simulink model "sim_qn6a"  (R2022b)
settings: Solver=ode4  StartTime=0.0  StopTime=8.0  FixedStep=tstep  RelTol=1e-3
undefined symbols (not defined in the file): den, num
settings Model: Creator=dipte  LastModifiedBy=dipte
settings DataIOCC: ReturnWorkspaceOutputs=off

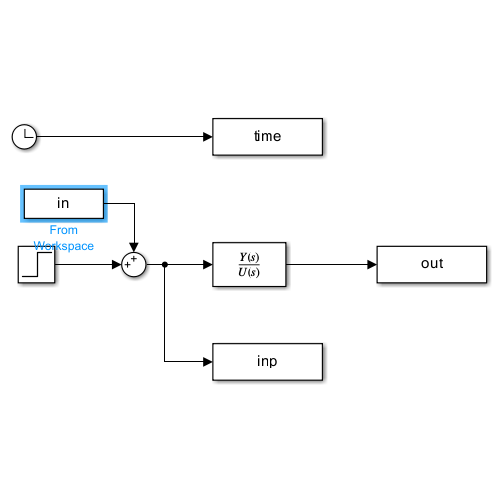
[thumbnail: Simulink's stored preview of the top-level diagram]
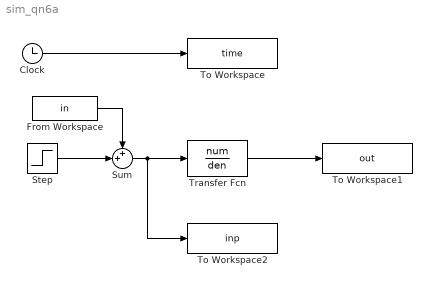
== system sim_qn6a ==
  Clock : Clock
  From Workspace : FromWorkspace  VariableName=in
  Step : Step  Time=0  SampleTime=0
  Sum : Sum  Inputs=++|
  To Workspace : ToWorkspace  VariableName=time  SampleTime=-1
      settings: Save2DSignal=2-D array (concatenate along first dimension)
  To Workspace1 : ToWorkspace  VariableName=out  SampleTime=-1
      settings: Save2DSignal=2-D array (concatenate along first dimension)
  To Workspace2 : ToWorkspace  VariableName=inp  SampleTime=-1
      settings: Save2DSignal=2-D array (concatenate along first dimension)
  Transfer Fcn : TransferFcn  Numerator=num  Denominator=den
  wires:
  Clock/1 -> To Workspace/1
  Transfer Fcn/1 -> To Workspace1/1
  Sum/1 -> To Workspace2/1, Transfer Fcn/1
  Step/1 -> Sum/2
  From Workspace/1 -> Sum/1
